simulink model "Motor"  (R2018b)
settings: Solver=VariableStepAuto  StartTime=0.0  StopTime=10.0  RelTol=1e-3
values from neighbouring files (symbols this model uses):
  efficiency_table = [85 85 85 85 85 85 85 85 85 85 85 85 85 85 85;85 85 85 85 85 85 85 85 85 85 85 85 85 85 85;85 85 90 90 90 90 90 90 90 90 88 88 88 88 88;85 85 92 92 92 92 92 92 92 92 92 90 90 90 90;85 85 92 92 93 93 93 93 92 92 92 90 90 90 90;85 85 93 94 94 94 94 94 94 94 94 94 94 94 94;85 85 93 94 94 95 95 95 95 95 95 95 95 95 95;85 85 93 94 94 95 95 95 95 95 95 95 95 95 95;85 85 93 94 95 95 95 95 95 95 95 95 95  ...(+141 chars)    [Motor.m]
  power_max = 80000    [Motor.m]
  T_eff_bp = [0 20 40 60 80 100 120 140 160 180 200 220 240 260 280]    [Motor.m]
  Tc = 0.02    [Motor.m]
  torque_max = 280    [Motor.m]
  w_eff_bp = [0 1000 2000 2728.370453 3000 4000 5000 6000 7000 8000 9000 10000]    [Motor.m]
libraries: autolibmappedmotorcommon x2
settings Model: Creator=xiaom  LastModifiedBy=xiaom

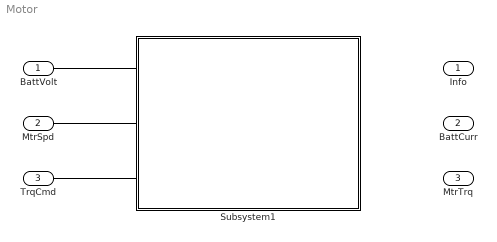
== system Motor ==
  BattVolt : Inport
  MtrSpd : Inport  Port=2
  TrqCmd : Inport  Port=3
  Subsystem1 : Subsystem
  Info : Outport
  BattCurr : Outport  Port=2
  MtrTrq : Outport  Port=3
  wires:
  ? -> MtrTrq/1
  ? -> BattCurr/1
  ? -> Info/1
  BattVolt/1 -> ?
  MtrSpd/1 -> ?
  TrqCmd/1 -> ?

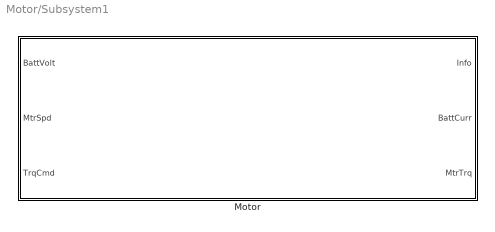
== system Motor/Subsystem1 ==
  Motor : Subsystem

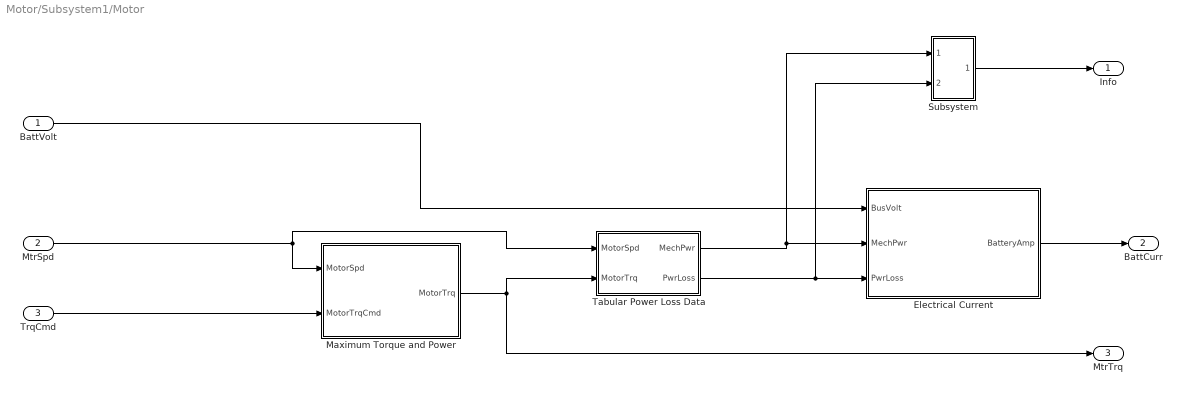
== system Motor/Subsystem1/Motor ==
  BattVolt : Inport  Unit=V
  MtrSpd : Inport  Port=2  Unit=rad/s
  TrqCmd : Inport  Port=3  Unit=N*m
  Electrical Current : Subsystem
  "Maximum Torque and Power " : Subsystem
  Subsystem : Subsystem
  Tabular Power Loss Data : Subsystem
  Info : Outport
  BattCurr : Outport  Port=2  Unit=A
  MtrTrq : Outport  Port=3  Unit=N*m
  wires:
  Subsystem/1(Info) -> Info/1
  MtrSpd/1 -> Tabular Power Loss Data/1(MotorSpd), "Maximum Torque and Power "/1(MotorSpd)
  Tabular Power Loss Data/1(MechPwr) -> Subsystem/1(MechPwr), Electrical Current/2(MechPwr)
  "Maximum Torque and Power "/1(MotorTrq) -> MtrTrq/1, Tabular Power Loss Data/2(MotorTrq)
  Tabular Power Loss Data/2(PwrLoss) -> Subsystem/2(PwrLoss), Electrical Current/3(PwrLoss)
  TrqCmd/1 -> "Maximum Torque and Power "/2(MotorTrqCmd)
  BattVolt/1 -> Electrical Current/1(BusVolt)
  Electrical Current/1(BatteryAmp) -> BattCurr/1

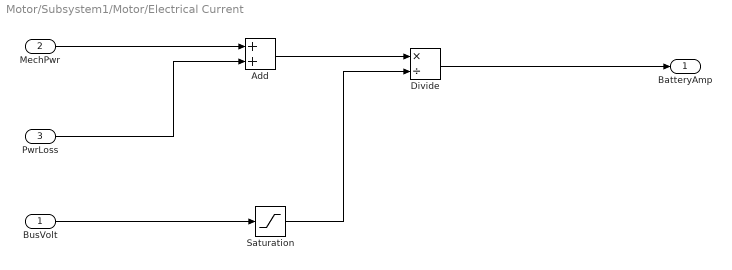
== system Motor/Subsystem1/Motor/Electrical Current ==
  BusVolt : Inport
  MechPwr : Inport  Port=2
  PwrLoss : Inport  Port=3
  Add : Sum
  Divide : Product  Inputs=*/
  Saturation : Saturate  UpperLimit=Inf  LowerLimit=0.0001
  BatteryAmp : Outport
  wires:
  Add/1 -> Divide/1
  Divide/1 -> BatteryAmp/1
  Saturation/1 -> Divide/2
  MechPwr/1 -> Add/1
  PwrLoss/1 -> Add/2
  BusVolt/1 -> Saturation/1

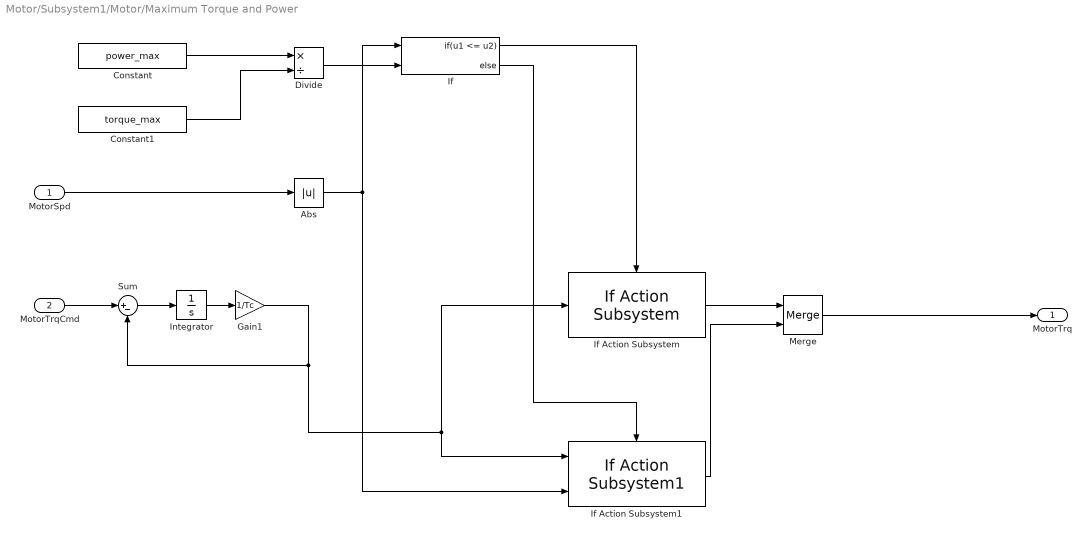
== system Motor/Subsystem1/Motor/Maximum Torque and Power  ==
  MotorSpd : Inport
  MotorTrqCmd : Inport  Port=2
  Abs : Abs
  Constant : Constant  Value=power_max
  Constant1 : Constant  Value=torque_max
  Divide : Product  Inputs=*/
  Gain1 : Gain  Gain=1/Tc
  If : If  NumInputs=2  IfExpression=u1 <= u2
  If Action Subsystem : autolibmappedmotorcommon/Maximum Torque and Power/If Action Subsystem  SystemSampleTime=-1
      settings: SourceProductName=Powertrain Blockset  SourceProductBaseCode=PW
  If Action Subsystem1 : autolibmappedmotorcommon/Maximum Torque and Power/If Action Subsystem1  SystemSampleTime=-1
      settings: SourceProductName=Powertrain Blockset  SourceProductBaseCode=PW
  Integrator : Integrator
  Merge : Merge  InitialOutput=0
  Sum : Sum  Inputs=|+-
  MotorTrq : Outport
  wires:
  Gain1/1 -> Sum/2, If Action Subsystem1/1, If Action Subsystem/1
  If/1 -> If Action Subsystem/Action
  Constant/1 -> Divide/1
  MotorTrqCmd/1 -> Sum/1
  MotorSpd/1 -> Abs/1
  Constant1/1 -> Divide/2
  Integrator/1 -> Gain1/1
  Divide/1 -> If/2
  If Action Subsystem1/1 -> Merge/2
  Merge/1 -> MotorTrq/1
  Sum/1 -> Integrator/1
  Abs/1 -> If Action Subsystem1/2, If/1
  If/2 -> If Action Subsystem1/Action
  If Action Subsystem/1 -> Merge/1

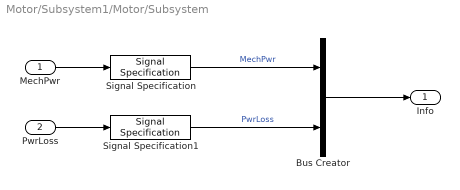
== system Motor/Subsystem1/Motor/Subsystem ==
  MechPwr : Inport
  PwrLoss : Inport  Port=2
  Bus Creator : BusCreator  Inputs=2
  Signal Specification : SignalSpecification  Unit=W
  Signal Specification1 : SignalSpecification  Unit=W
  Info : Outport
  wires:
  Signal Specification/1 -> Bus Creator/1  "MechPwr"
  Signal Specification1/1 -> Bus Creator/2  "PwrLoss"
  MechPwr/1 -> Signal Specification/1
  Bus Creator/1 -> Info/1
  PwrLoss/1 -> Signal Specification1/1

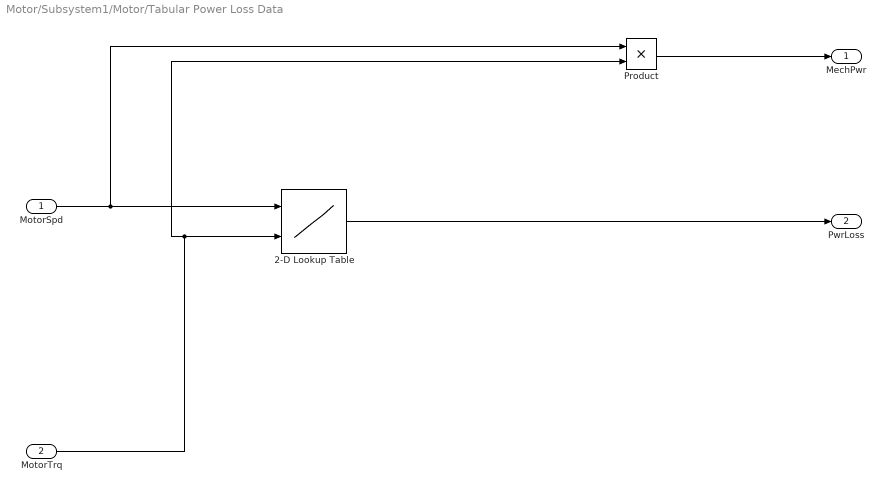
== system Motor/Subsystem1/Motor/Tabular Power Loss Data ==
  MotorSpd : Inport
  MotorTrq : Inport  Port=2
  2-D Lookup Table : Lookup_n-D  BreakpointsForDimension1=w_eff_bp  BreakpointsForDimension2=T_eff_bp  Table=efficiency_table  ExtrapMethod=Clip  UseLastTableValue=on  InternalRulePriority=Speed  RndMeth=Simplest  InputSameDT=on
  Product : Product
  MechPwr : Outport
  PwrLoss : Outport  Port=2
  wires:
  MotorTrq/1 -> Product/2, 2-D Lookup Table/2
  Product/1 -> MechPwr/1
  2-D Lookup Table/1 -> PwrLoss/1
  MotorSpd/1 -> 2-D Lookup Table/1, Product/1
